simulink model "Temporal1_2018a"  (R2018a)
settings: Solver=VariableStepAuto  StartTime=0.0  StopTime=1.0  RelTol=1e-3
settings Model: Creator=86188  LastModifiedBy=bzhan

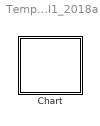
== system Temporal1_2018a ==
  Chart : Stateflow chart  TreatAsAtomicUnit=on

== stateflow chart Temporal1_2018a/Chart ==
  settings: updateMethod=DISCRETE  sampleTime=0.1
  state A
    en:f("en_A");
    du:f("du_A");
  state B
    en:f("en_B")
    du:f("du_B");
  (default) -> A
  A -> B : after(3,tick)
  B -> A : after(3,tick)
  data: s function_input
  function f(s):
    | function f(s)
    |   fprintf(s+"\n");
